simulink model "SimpleAcquisition_16ch_2014a_RT_preProc"  (R2014a)
settings: Solver=FixedStepDiscrete  StartTime=0.0  StopTime=inf  FixedStep=1/512  RelTol=1e-3
StartFcn:
  | simulinkModelStartFcn('SimpleAcquisition_16ch_2014a_RT_preProc')
undefined symbols (not defined in the file or in its folder): currentCFG_SimpleAcquisition_16ch_2014a_RT_preProc_UB, UB
libraries: dspsigattribs x1, Tools x1, gtecHighspeedLib x1, gUSBamplib x1
settings Model: Creator=Leonardo  LastModifiedBy=Leonardo
settings DebuggingCC: MergeDetectMultiDrivingBlocksExec=error  FrameProcessingCompatibilityMsg=error

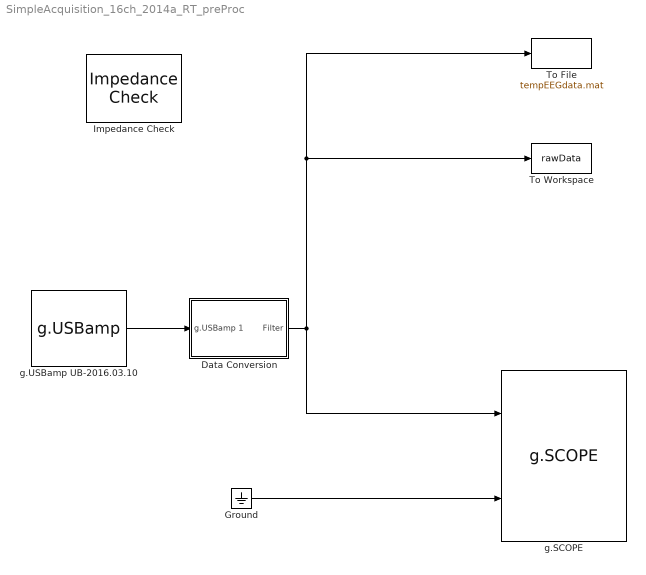
== system SimpleAcquisition_16ch_2014a_RT_preProc ==
  "Data Conversion " : Subsystem
  Ground : Ground
  Impedance Check : Tools/Impedance Check
  To File : ToFile  Filename=tempEEGdata.mat  SaveFormat=Timeseries
  To Workspace : ToWorkspace  VariableName=rawData  SaveFormat=Timeseries  SampleTime=-1
  g.SCOPE : gtecHighspeedLib/g.SCOPE
  g.USBamp UB-2016.03.10 : gUSBamplib/g.USBamp  Priority=1  cfg=currentCFG_SimpleAcquisition_16ch_2014a_RT_preProc_UB-2016.03.10.cfg  snr=UB-2016.03.10
  wires:
  Ground/1 -> g.SCOPE/2
  "Data Conversion "/1(Filter) -> To File/1, To Workspace/1, g.SCOPE/1
  g.USBamp UB-2016.03.10/1 -> "Data Conversion "/1(g.USBamp 1)

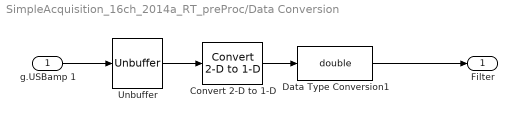
== system SimpleAcquisition_16ch_2014a_RT_preProc/Data Conversion  ==
  g.USBamp 1 : Inport  Priority=2
  Convert 2-D to 1-D : dspsigattribs/Convert 2-D to 1-D
  Data Type Conversion1 : DataTypeConversion  OutDataTypeStr=double
  Unbuffer : Unbuffer  SampleBasedProcessing=Same as frame based
  Filter : Outport
  wires:
  g.USBamp 1/1 -> Unbuffer/1
  Unbuffer/1 -> Convert 2-D to 1-D/1
  Convert 2-D to 1-D/1 -> Data Type Conversion1/1
  Data Type Conversion1/1 -> Filter/1
